simulink subsystem "aeroForcesCalculation"  (R2025b)
settings: Solver=VariableStepAuto  StartTime=0.0  StopTime=10.0  RelTol=1e-3
values from neighbouring files (symbols this model uses):
  vehicleParams = 18.0    [plantParams.sldd]
libraries: matrix_library x1, vrlib x1
settings Model: Creator=maxhu  LastModifiedBy=mowen25

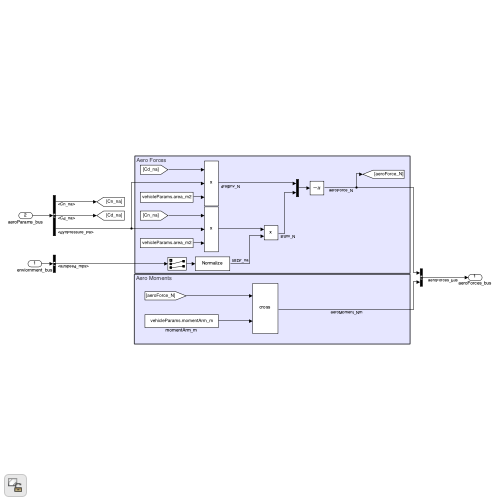
[thumbnail: Simulink's stored preview of the top-level diagram]
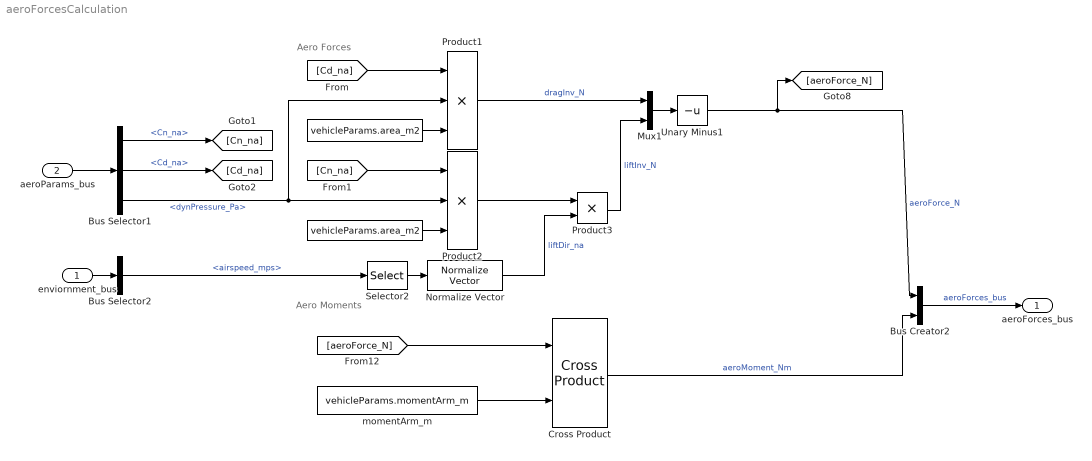
== system aeroForcesCalculation ==
  note: Aero Moments
  note: Aero Forces
  enviornment_bus : Inport
  aeroParams_bus : Inport  Port=2
  " " : Constant  Value=vehicleParams.area_m2
  "   " : Constant  Value=vehicleParams.area_m2
  Bus Creator2 : BusCreator  Inputs=2
  Bus Selector1 : BusSelector  OutputSignals=Cn_na,Cd_na,dynPressure_Pa
  Bus Selector2 : BusSelector  OutputSignals=airspeed_mps
  Cross Product : matrix_library/Cross Product
  Mux1 : Mux  Inputs=2
  Normalize Vector : vrlib/Utilities/Normalize Vector  maxzero=0
  Product1 : Product  Inputs=3
  Product2 : Product  Inputs=3
  Product3 : Product
  Selector2 : Selector  InputPortWidth=3  IndexOptions=Index vector (dialog)  Indices=[2 3]  OutputSizes=1
  Unary Minus1 : UnaryMinus
  momentArm_m : Constant  Value=vehicleParams.momentArm_m
  aeroForces_bus : Outport
  wires:
  Normalize Vector/1 -> Product3/2  "liftDir_na"
  Cross Product/1 -> Bus Creator2/2  "aeroMoment_Nm"
  [aeroForce_N] -> Cross Product/1
  " "/1 -> Product2/3
  Product3/1 -> Mux1/2  "liftInv_N"
  Mux1/1 -> Unary Minus1/1
  Unary Minus1/1 -> [aeroForce_N], Bus Creator2/1  "aeroForce_N"
  Selector2/1 -> Normalize Vector/1
  Product1/1 -> Mux1/1  "dragInv_N"
  momentArm_m/1 -> Cross Product/2
  Product2/1 -> Product3/1
  Bus Selector2/1 -> Selector2/1  "<airspeed_mps>"
  enviornment_bus/1 -> Bus Selector2/1
  Bus Creator2/1 -> aeroForces_bus/1  "aeroForces_bus"
  aeroParams_bus/1 -> Bus Selector1/1
  Bus Selector1/2 -> [Cd_na]  "<Cd_na>"
  Bus Selector1/1 -> [Cn_na]  "<Cn_na>"
  Bus Selector1/3 -> Product2/2, Product1/2  "<dynPressure_Pa>"
  [Cd_na] -> Product1/1
  [Cn_na] -> Product2/1
  "   "/1 -> Product1/3
